simulink model "pb3"  (R2020b)
settings: Solver=VariableStepAuto  StartTime=0.0  StopTime=10.0  RelTol=1e-3
settings Model: Creator=Shivani  LastModifiedBy=Shivani

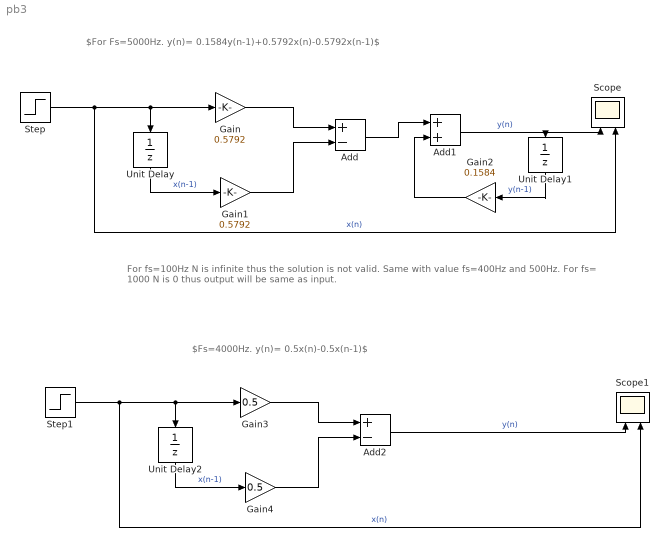
== system pb3 ==
  note: $For Fs=5000Hz. y(n)= 0.1584y(n-1)+0.5792x(n)-0.5792x(n-1)$
  note: For fs=100Hz N is infinite thus the solution is not valid. Same with value fs=400Hz and 500Hz. For fs= 1000 N is 0 thus output will be same as input.
  note: $Fs=4000Hz. y(n)= 0.5x(n)-0.5x(n-1)$
  Add : Sum  Inputs=+-
  Add1 : Sum
  Add2 : Sum  Inputs=+-
  Gain : Gain  Gain=0.5792
  Gain1 : Gain  Gain=0.5792
  Gain2 : Gain  Gain=0.1584
  Gain3 : Gain  Gain=0.5
  Gain4 : Gain  Gain=0.5
  Scope : Scope  NumInputPorts=2
  Scope1 : Scope  NumInputPorts=2
  Step : Step  SampleTime=0
  Step1 : Step  SampleTime=0
  Unit Delay : UnitDelay  SampleTime=-1  HasFrameUpgradeWarning=on
  Unit Delay1 : UnitDelay  SampleTime=-1  HasFrameUpgradeWarning=on
  Unit Delay2 : UnitDelay  SampleTime=-1  HasFrameUpgradeWarning=on
  wires:
  Gain1/1 -> Add/2
  Step/1 -> Gain/1, Unit Delay/1, Scope/2  "x(n)"
  Unit Delay1/1 -> Gain2/1  "y(n-1)"
  Unit Delay/1 -> Gain1/1  "x(n-1)"
  Gain2/1 -> Add1/2
  Gain/1 -> Add/1
  Add/1 -> Add1/1
  Add1/1 -> Scope/1, Unit Delay1/1  "y(n)"
  Unit Delay2/1 -> Gain4/1  "x(n-1)"
  Step1/1 -> Gain3/1, Unit Delay2/1, Scope1/2  "x(n)"
  Gain4/1 -> Add2/2
  Gain3/1 -> Add2/1
  Add2/1 -> Scope1/1  "y(n)"
